simulink model "shape_delay_atten"  (R2020b)
settings: Solver=VariableStepAuto  StartTime=0.0  StopTime=10.0  RelTol=1e-3
values from neighbouring files (symbols this model uses):
  t_delay = shaper_struct.t_delay;'    [sim_shaper.m]    (also in zz_cfd.m = 500e-12;'; zz_noShape.m = 1.337e-08)
  v_LED = .02    (= 0.02)    [zz_cfd.m]
undefined symbols (not defined in the file or in its folder): f_attenuation
libraries: simulink x2
settings Model: Creator=lydialee  LastModifiedBy=lydialee

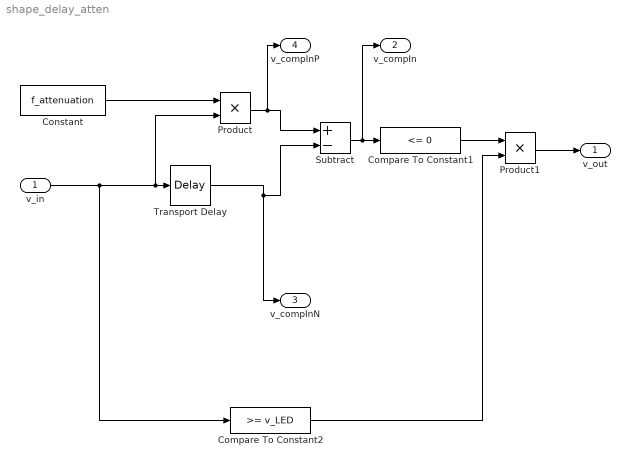
== system shape_delay_atten ==
  v_in : Inport
  Compare To Constant1 : simulink/Logic and Bit Operations/Compare To Constant  relop=<=  const=0  OutDataTypeStr=boolean
  Compare To Constant2 : simulink/Logic and Bit Operations/Compare To Constant  relop=>=  const=v_LED  OutDataTypeStr=boolean
  Constant : Constant  Value=f_attenuation
  Product : Product
  Product1 : Product
  Subtract : Sum  Inputs=+-
  Transport Delay : TransportDelay  DelayTime=t_delay
  v_out : Outport  VectorParamsAs1DForOutWhenUnconnected=off
  v_compIn : Outport  Port=2  VectorParamsAs1DForOutWhenUnconnected=off
  v_compInN : Outport  Port=3  VectorParamsAs1DForOutWhenUnconnected=off
  v_compInP : Outport  Port=4  VectorParamsAs1DForOutWhenUnconnected=off
  wires:
  Transport Delay/1 -> v_compInN/1, Subtract/2
  Subtract/1 -> v_compIn/1, Compare To Constant1/1
  v_in/1 -> Compare To Constant2/1, Transport Delay/1, Product/2
  Constant/1 -> Product/1
  Product/1 -> v_compInP/1, Subtract/1
  Compare To Constant2/1 -> Product1/2
  Compare To Constant1/1 -> Product1/1
  Product1/1 -> v_out/1
